simulink library "moneylib"  (Simulink 8.6)
settings: Solver=VariableStepAuto  SolverMode=SingleTasking  StartTime=0.0  StopTime=10.0  RelTol=1e-3
settings Model: Creator=gcampa  LastModifiedBy=gcampa

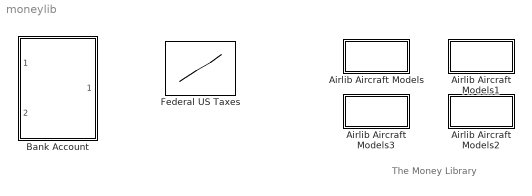
== system moneylib ==
  note: The Money Library
  Airlib Aircraft Models : Subsystem
      settings: OpenFcn=tax_block_example
      mask Display: disp('Tax Block\nExample')
  Airlib Aircraft Models1 : Subsystem
      settings: OpenFcn=bank_block_example
      mask Display: disp('Bank Block\nExample')
  Airlib Aircraft Models2 : Subsystem
      settings: OpenFcn=DistributionFlow
      mask Display: disp('Distribution\nFlow')
  Airlib Aircraft Models3 : Subsystem
      settings: OpenFcn=ContributionFlow
      mask Display: disp('Contribution\nFlow')
  Bank Account : Subsystem  mask(Bank Account){i=0.03, j=0.01, x0=0}
      mask prompts: i "Interest rate"; j "Inflation"; x0 "Initial Amount"
      mask help: Deposits and Expenses are given as first and second input, respectively. The expense amount is multiplied by (1+j)^k to account for inflation and the result is subtracted from the deposit to determine the amount that stays in the bank and earns interests after each period. The output of the block is the money available at the current time. Look under the mask for more insights.
      mask Help:
      | Deposits and Expenses are given as first and second input, respectively.
      | The expense amount is multiplied by (1+j)^k to account for inflation and the result is subtracted from the deposit to determine the amount that stays in the bank, and earns interests after each period.
      | The output of the block is the money available at the current time.
      | Look under the mask for more insights.
  Federal US Taxes : Lookup_n-D  NumberOfTableDimensions=1  BreakpointsForDimension1=xT  Table=yT  InternalRulePriority=Speed  RndMeth=Simplest  InputSameDT=on  mask(Taxes Look Up table){x=[9875 40125 85525 163300 207350 518400], p=[0.10 0.12 0.22 0.24 0.32 0.35 0.37]}
      mask prompts: x "Bracket upper limits"; p "Bracket tax rates"
      mask help:
      | This block calculates the taxes due for a given yearly income, according to a given progressive tax bracket system.
      | The input is the yearly income, the output is the tax amount due. The bracket upper limits and rates are the two mask parameter.
      | The first rate applies to income below the first upper limit and the last rate applies for incomes above the last upper limit.
      mask init:
      | xT=[0,x(:)',2*x(end)];
      | yT=0; for i=1:length(xT)-1, yT(i+1)=yT(i)+(xT(i+1)-xT(i))*p(i); end
      mask Help:
      | This block calculates the taxes due for a given yearly income, according to a given progressive tax bracket system.
      | The input is the yearly income, the output is the tax amount due.
      | The bracket upper limits and rates are the two mask parameter.
      | The first rate applies to income below the first upper limit and the last rate applies for incomes above the last upper limit.
      | 2020 Tax brackets are taken from: https://taxfoundation.org/2020-tax-brackets/
      | See also the function taxes.m in the "others" folder, which uses an additive algorithm to return the same result (for positive inputs).

== system moneylib/Airlib Aircraft Models ==

== system moneylib/Airlib Aircraft Models1 ==

== system moneylib/Airlib Aircraft Models2 ==

== system moneylib/Airlib Aircraft Models3 ==

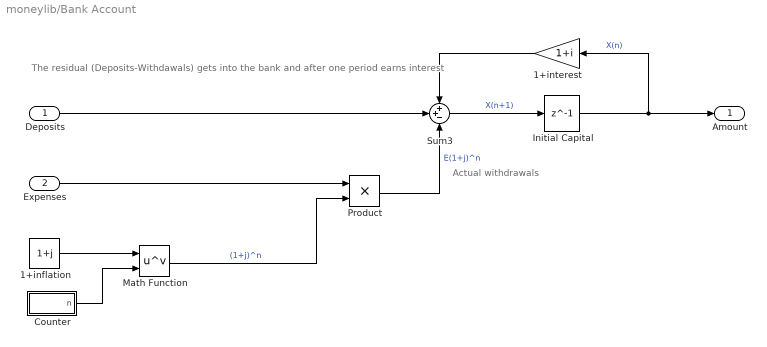
== system moneylib/Bank Account ==
  note: Actual
      | withdrawals
  note: The residual (Deposits-Withdawals) gets into the bank and after one period earns interest
  Deposits : Inport
  Expenses : Inport  Port=2
  1+inflation : Constant  Value=1+j
  1+interest : Gain  Gain=1+i
  Counter : Subsystem
  Initial Capital : Delay  DelayLength=1  InitialCondition=x0  SampleTime=1
  Math Function : Math  Operator=pow  SaturateOnIntegerOverflow=on
  Product : Product
  Sum3 : Sum  Inputs=++-
  Amount : Outport
  wires:
  1+interest/1 -> Sum3/1
  Initial Capital/1 -> Amount/1, 1+interest/1  "X(n)"
  1+inflation/1 -> Math Function/1
  Deposits/1 -> Sum3/2
  Expenses/1 -> Product/1
  Math Function/1 -> Product/2  "(1+j)^n"
  Product/1 -> Sum3/3  "E(1+j)^n"
  Sum3/1 -> Initial Capital/1  "X(n+1)"
  Counter/1(n) -> Math Function/2

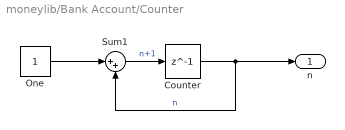
== system moneylib/Bank Account/Counter ==
  Counter : Delay  DelayLength=1  InitialCondition=0  SampleTime=1
  One : Constant
  Sum1 : Sum  Inputs=|++
  n : Outport
  wires:
  Sum1/1 -> Counter/1  "n+1"
  Counter/1 -> n/1, Sum1/2  "n"
  One/1 -> Sum1/1
